simulink model "Xcvr_SSB_AM_2p5"  (Simulink 8.0)
settings: Solver=VariableStepDiscrete  SolverMode=SingleTasking  StartTime=0.0  StopTime=10  RelTol=1e-3
PreLoadFcn:
  | Fs=80e6;
  | 
  | phee=da_rom();
  | [phee_1,phee_2]=da_i2_rom();
  | 
  | Dcic=64;       % CIC decimation
  | Dfac=128;    % following DA filter decimation
  | N = 6;           %       (2^(N+1))=Dfac
  | Daudio=Dcic*Dfac;
  | Faudio=Fs/Daudio;
  | 
  | load info_filt_ssb_4
  | load Serial_Intfc_Stream_5
  | 
  | % AGC related
  | x=0.5:1/256:(1-1/256);
  | addr=(x-0.5)*256;
  | y=1./x;
values from neighbouring files (symbols this model uses):
  Serial_Interface = [0 0 0 0 0 0 0 0 0 0 0 0 ... (11390 elements, 2x5695)]    [Serial_Intfc_Stream_5.mat]
undefined symbols (not defined in the file or in its folder): get, sided, Two, xlipgetpartsetting
undefined symbols (not defined in the file): ssb_coef
libraries: xbsIndex_r4 x1305, dspsrcs4 x5, simulink x2, dspsigops x2, dspsnks4 x1
(part 4 of 11)

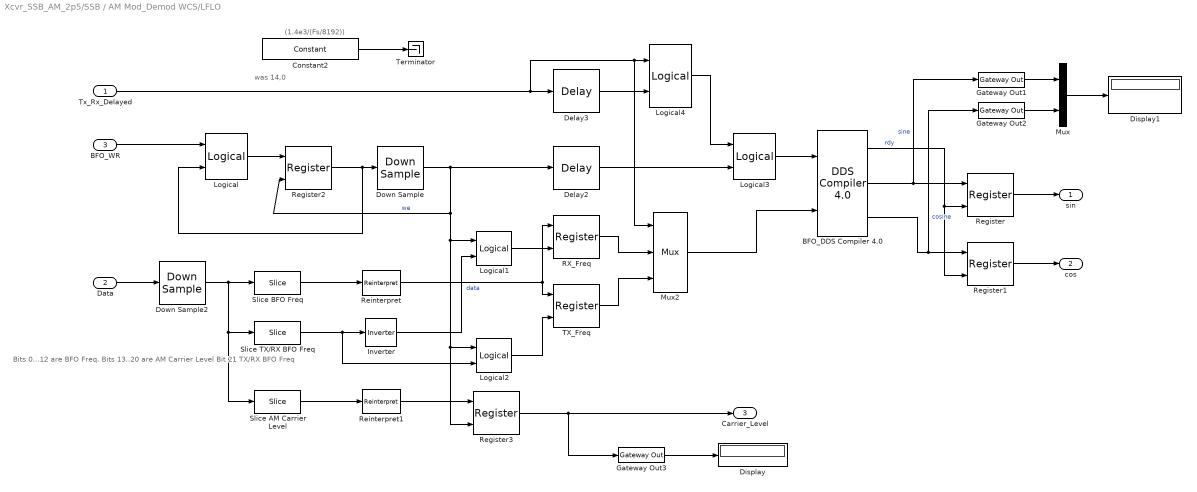
== system Xcvr_SSB_AM_2p5/SSB / AM Mod_Demod WCS/LFLO ==
  note: (1.4e3/(Fs/8192))
  note: was 14,0
  note: Bits 0...12  are BFO Freq.
      | Bits 13..20 are AM Carrier Level
      | Bit 21 TX/RX BFO Freq
  Tx_Rx_Delayed : Inport
  Data : Inport  Port=2
  BFO_WR : Inport  Port=3
  "BFO_DDS Compiler 4.0 " : xbsIndex_r4/DDS Compiler 4.0   partspresent=Phase_Generator_and_SIN_COS_LUT  dds_clock_rate="(Fs/4096)*1e-6 % a LIE  but 8192 does not work!!!!"  channels=1  parameter_entry=System_Parameters  spurious_free_dynamic_range=84  frequency_resolution=(Fs/Daudio)*2^-12  noise_shaping=Phase_Dithering  phase_width=28  output_width=6  output_selection=Sine_and_Cosine  negative_sine=off  negative_cosine=off  amplitude_mode=Full_Range  memory_type=Auto  optimization_goal=Area  dsp48_use=Minimal  latency_configuration=Auto  latency=2  has_phase_out=off  sclr_pin=off  clock_enable=off  rfd=off  rdy=on  channel_pin=off  explicit_period=off  period=1  phase_increment=Programmable  output_frequency1=0  output_frequency2=0  output_frequency3=0  output_frequency4=0  output_frequency5=0  output_frequency6=0  output_frequency7=0  output_frequency8=0  output_frequency9=0  output_frequency10=0  output_frequency11=0  output_frequency12=0  output_frequency13=0  output_frequency14=0  output_frequency15=0  output_frequency16=0  pinc1='0'  pinc2='0'  pinc3='0'  pinc4='0'  pinc5='0'  pinc6='0'  pinc7='0'  pinc8='0'  pinc9='0'  pinc10='0'  pinc11='0'  pinc12='0'  pinc13='0'  pinc14='0'  pinc15='0'  pinc16='0'  phase_offset=None  phase_offset_angles1=0  phase_offset_angles2=0  phase_offset_angles3=0  phase_offset_angles4=0  phase_offset_angles5=0  phase_offset_angles6=0  phase_offset_angles7=0  phase_offset_angles8=0  phase_offset_angles9=0  phase_offset_angles10=0  phase_offset_angles11=0  phase_offset_angles12=0  phase_offset_angles13=0  phase_offset_angles14=0  phase_offset_angles15=0  phase_offset_angles16=0  poff1='0'  poff2='0'  poff3='0'  poff4='0'  poff5='0'  poff6='0'  poff7='0'  poff8='0'  poff9='0'  poff10='0'  poff11='0'  poff12='0'  poff13='0'  poff14='0'  poff15='0'  poff16='0'  por_mode=false  gui_behaviour=Sysgen  ip_name=DDS Compiler  ip_version=4.0  dsptool_ready=true  wrapper_available=true  port_translation_map={ 'ce' => 'en', 'sclr' => 'rst' }  ipcore_xco_need_fpga_part=true  ipcore_fpga_part=xlipgetpartsetting(gcb, {'virtex4', 'xc4vsx35', '-10', 'ff668'})  ipcore_usecache=true  ipcore_useipmodelcache=true  ipcore_verbose=false  block_type=dds_compiler_v4_0
      settings: block_version=12.1
  Constant2 : xbsIndex_r4/Constant  const=(1.4e3/(Fs/8192))  gui_display_data_type=Fixed-point  arith_type=Signed (2's comp)  n_bits=13  bin_pt=13  preci_type=Single  exp_width=8  frac_width=24  explicit_period=on  period=8192/Fs  equ=P=C  opselect=C  inp2=PCIN>>17  opr=+  inp1=P  carry=CIN  dbl_ovrd=off  block_type=constant
      settings: block_version=9.2.00
  Delay2 : xbsIndex_r4/Delay  rst=off  infoeditControl=Selection of Reset will increase slice count due to use of real FFs and instead of SRLs  en=off  latency=1  dbl_ovrd=off  reg_retiming=off  block_type=delay
      settings: block_version=12.1
  Delay3 : xbsIndex_r4/Delay  rst=off  infoeditControl=Selection of Reset will increase slice count due to use of real FFs and instead of SRLs  en=off  latency=1  dbl_ovrd=off  reg_retiming=off  block_type=delay
      settings: block_version=12.1
  Display : Display
  Display1 : Display
  Down Sample : xbsIndex_r4/Down Sample  sample_ratio=1024  sample_phase=First Value of Frame  en=off  latency=0  dbl_ovrd=off  block_type=dsamp
      settings: block_version=9.2.00
  Down Sample2 : xbsIndex_r4/Down Sample  sample_ratio=1024  sample_phase=First Value of Frame  en=off  latency=0  dbl_ovrd=off  block_type=dsamp
      settings: block_version=9.2.00
  Gateway Out1 : xbsIndex_r4/Gateway Out  inherit_from_input=off  hdl_port=off  timing_constraint=None  locs_specified=off  LOCs={}  UseAsDAC=off  DACChannel='1'  block_type=gatewayout
      settings: infoedit="Gateway out block.  Converts Xilinx fixed point inputs into ouputs of type Simulink integer, double, or fixed point.<P><P>Hardware notes:  In hardware these blocks become top level output ports or are discarded, depending on how they are configured."  block_version=9.2.00
  Gateway Out2 : xbsIndex_r4/Gateway Out  inherit_from_input=off  hdl_port=off  timing_constraint=None  locs_specified=off  LOCs={}  UseAsDAC=off  DACChannel='1'  block_type=gatewayout
      settings: infoedit="Gateway out block.  Converts Xilinx fixed point inputs into ouputs of type Simulink integer, double, or fixed point.<P><P>Hardware notes:  In hardware these blocks become top level output ports or are discarded, depending on how they are configured."  block_version=9.2.00
  Gateway Out3 : xbsIndex_r4/Gateway Out  inherit_from_input=off  hdl_port=off  timing_constraint=None  locs_specified=off  LOCs={}  UseAsDAC=off  DACChannel='1'  block_type=gatewayout
      settings: infoedit="Gateway out block.  Converts Xilinx fixed point inputs into ouputs of type Simulink integer, double, or fixed point.<P><P>Hardware notes:  In hardware these blocks become top level output ports or are discarded, depending on how they are configured."  block_version=9.2.00
  Inverter : xbsIndex_r4/Inverter  en=off  latency=0  dbl_ovrd=off  block_type=inv
      settings: block_version=12.2
  Logical : xbsIndex_r4/Logical  logical_function=OR  inputs=2  en=off  latency=0  precision=Full  arith_type=Unsigned  n_bits=16  bin_pt=0  align_bp=on  dbl_ovrd=off  block_type=logical
      settings: block_version=9.2.00
  Logical1 : xbsIndex_r4/Logical  logical_function=AND  inputs=2  en=off  latency=0  precision=Full  arith_type=Unsigned  n_bits=16  bin_pt=0  align_bp=on  dbl_ovrd=off  block_type=logical
      settings: block_version=12.2
  Logical2 : xbsIndex_r4/Logical  logical_function=AND  inputs=2  en=off  latency=0  precision=Full  arith_type=Unsigned  n_bits=16  bin_pt=0  align_bp=on  dbl_ovrd=off  block_type=logical
      settings: block_version=12.2
  Logical3 : xbsIndex_r4/Logical  logical_function=OR  inputs=2  en=off  latency=0  precision=Full  arith_type=Unsigned  n_bits=16  bin_pt=0  align_bp=on  dbl_ovrd=off  block_type=logical
      settings: block_version=12.1
  Logical4 : xbsIndex_r4/Logical  logical_function=XOR  inputs=2  en=off  latency=0  precision=Full  arith_type=Unsigned  n_bits=16  bin_pt=0  align_bp=on  dbl_ovrd=off  block_type=logical
      settings: block_version=12.1
  Mux : Mux  Inputs=2
  Mux2 : xbsIndex_r4/Mux  inputs=2  en=off  latency=0  precision=Full  arith_type=Unsigned  n_bits=16  bin_pt=14  quantization=Truncate  overflow=Wrap  dbl_ovrd=off  block_type=mux
      settings: block_version=12.1
  RX_Freq : xbsIndex_r4/Register  init=0  rst=off  en=on  dbl_ovrd=off  block_type=register
      settings: block_version=12.1
  Register : xbsIndex_r4/Register  init=0  rst=off  en=on  dbl_ovrd=off  block_type=register
      settings: block_version=9.2.00
  Register1 : xbsIndex_r4/Register  init=0  rst=off  en=on  dbl_ovrd=off  block_type=register
      settings: block_version=9.2.00
  Register2 : xbsIndex_r4/Register  init=0  rst=on  en=off  dbl_ovrd=off  block_type=register
      settings: block_version=9.2.00
  Register3 : xbsIndex_r4/Register  init=0.5  rst=off  en=on  dbl_ovrd=off  block_type=register
      settings: block_version=9.2.00
  Reinterpret : xbsIndex_r4/Reinterpret  force_arith_type=on  arith_type="Signed  (2's comp)"  force_bin_pt=on  bin_pt=13  block_type=reinterpret
      settings: infoedit="Changes signal type without altering the binary representation.   You can changed the signal between signed and unsigned, and relocate the binary point.<br><br>Hardware notes: In hardware this block costs nothing.<br><br>Example:  Suppose the input is 6 bits wide, signed, with 2 fractional bits, and the output is forced to unsigned with 0 fractional bits.  Then an input of -2.0 (1110.00 in binary 2's complement) becomes an output of 56 (111000 in binary)."  block_version=9.2.00
  Reinterpret1 : xbsIndex_r4/Reinterpret  force_arith_type=on  arith_type=Unsigned  force_bin_pt=on  bin_pt=8  block_type=reinterpret
      settings: infoedit="Changes signal type without altering the binary representation.   You can changed the signal between signed and unsigned, and relocate the binary point.<br><br>Hardware notes: In hardware this block costs nothing.<br><br>Example:  Suppose the input is 6 bits wide, signed, with 2 fractional bits, and the output is forced to unsigned with 0 fractional bits.  Then an input of -2.0 (1110.00 in binary 2's complement) becomes an output of 56 (111000 in binary)."  block_version=9.2.00
  Slice AM Carrier Level : xbsIndex_r4/Slice  nbits=8  boolean_output=off  mode=Lower Bit Location + Width  bit1=0  base1=MSB of Input  bit0=13  base0=LSB of Input  dbl_ovrd=off  block_type=slice
      settings: block_version=9.2.00
  Slice BFO Freq : xbsIndex_r4/Slice  nbits=13  boolean_output=off  mode=Lower Bit Location + Width  bit1=0  base1=MSB of Input  bit0=0  base0=LSB of Input  dbl_ovrd=off  block_type=slice
      settings: block_version=9.2.00
  Slice TX/RX BFO Freq : xbsIndex_r4/Slice  nbits=1  boolean_output=on  mode=Lower Bit Location + Width  bit1=0  base1=MSB of Input  bit0=21  base0=LSB of Input  dbl_ovrd=off  block_type=slice
      settings: block_version=9.2.00
  TX_Freq : xbsIndex_r4/Register  init=0  rst=off  en=on  dbl_ovrd=off  block_type=register
      settings: block_version=12.1
  Terminator : Terminator
  sin : Outport
  cos : Outport  Port=2
  Carrier_Level : Outport  Port=3
  wires:
  BFO_WR/1 -> Logical/1
  Register/1 -> sin/1
  Register1/1 -> cos/1
  Constant2/1 -> Terminator/1
  Slice BFO Freq/1 -> Reinterpret/1
  Down Sample/1 -> Delay2/1, Register2/2, Logical1/1, Register3/2, Logical2/1  "we"
  Logical/1 -> Register2/1
  Register2/1 -> Logical/2, Down Sample/1
  Gateway Out3/1 -> Display/1
  Data/1 -> Down Sample2/1
  "BFO_DDS Compiler 4.0 "/1 -> Register1/2, Register/2  "rdy"
  "BFO_DDS Compiler 4.0 "/2 -> Register/1, Gateway Out1/1  "sine"
  "BFO_DDS Compiler 4.0 "/3 -> Register1/1, Gateway Out2/1  "cosine"
  Gateway Out1/1 -> Mux/1
  Gateway Out2/1 -> Mux/2
  Mux/1 -> Display1/1
  Slice AM Carrier Level/1 -> Reinterpret1/1
  Reinterpret1/1 -> Register3/1
  Register3/1 -> Carrier_Level/1, Gateway Out3/1
  Down Sample2/1 -> Slice BFO Freq/1, Slice AM Carrier Level/1, Slice TX/RX BFO Freq/1
  Logical3/1 -> "BFO_DDS Compiler 4.0 "/1
  Delay3/1 -> Logical4/2
  Logical4/1 -> Logical3/1
  Delay2/1 -> Logical3/2
  Tx_Rx_Delayed/1 -> Delay3/1, Logical4/1, Mux2/1
  RX_Freq/1 -> Mux2/2
  TX_Freq/1 -> Mux2/3
  Mux2/1 -> "BFO_DDS Compiler 4.0 "/2
  Reinterpret/1 -> RX_Freq/1, TX_Freq/1  "data"
  Slice TX/RX BFO Freq/1 -> Inverter/1, Logical2/2
  Logical1/1 -> RX_Freq/2
  Inverter/1 -> Logical1/2
  Logical2/1 -> TX_Freq/2

== system Xcvr_SSB_AM_2p5/SSB / AM Mod_Demod WCS/Sequential_Complex_abs() ==
  note: Fixed Point Iterative Square Root with Pre/Post Scaling
  In_I : Inport
  In_Q : Inport  Port=2
  AddSub : xbsIndex_r4/AddSub  mode=Addition  use_carryin=off  use_carryout=off  en=off  latency=0  precision=User Defined  arith_type=Unsigned  n_bits=32  bin_pt=31  quantization=Truncate  overflow=Saturate  dbl_ovrd=off  use_behavioral_HDL=off  hw_selection=Fabric  pipelined=off  block_type=addsub
      settings: block_version=12.1
  Convert NOTE Rounding : xbsIndex_r4/Convert  gui_display_data_type=Fixed-point  arith_type="Signed  (2's comp)"  n_bits=18  bin_pt=17  float_type=Single  exp_bits=8  fraction_bits=24  quantization="Round  (unbiased: +/- Inf)"  overflow=Saturate  en=off  latency=0  dbl_ovrd=off  pipeline=off  block_type=convert
      settings: block_version=12.1
  Convert NOTE Rounding1 : xbsIndex_r4/Convert  gui_display_data_type=Fixed-point  arith_type=Unsigned  n_bits=16  bin_pt=15  float_type=Single  exp_bits=8  fraction_bits=24  quantization="Round  (unbiased: +/- Inf)"  overflow=Wrap  en=off  latency=1  dbl_ovrd=off  pipeline=off  block_type=convert
      settings: block_version=12.1
  Delay : xbsIndex_r4/Delay  rst=off  infoeditControl=Selection of Reset will increase slice count due to use of real FFs and instead of SRLs  en=off  latency=1  dbl_ovrd=off  reg_retiming=off  block_type=delay
      settings: block_version=12.1
  Delay1 : xbsIndex_r4/Delay  rst=off  infoeditControl=Selection of Reset will increase slice count due to use of real FFs and instead of SRLs  en=off  latency=1  dbl_ovrd=off  reg_retiming=off  block_type=delay
      settings: block_version=12.1
  Down Sample : xbsIndex_r4/Down Sample  sample_ratio=32  sample_phase="Last Value of Frame  (most efficient)"  en=off  latency=1  dbl_ovrd=off  block_type=dsamp
      settings: block_version=12.1
  Iterative SQRT : Subsystem
  Pre Scaler : Subsystem
  Sequential Post Scale : Subsystem
  Time Shared Square Operator : Subsystem
  Up Sample : xbsIndex_r4/Up Sample  sample_ratio=32  copy_samples=on  en=off  latency=0  dbl_ovrd=off  block_type=usamp
      settings: block_version=12.1
  Up Sample1 : xbsIndex_r4/Up Sample  sample_ratio=32  copy_samples=on  en=off  latency=0  dbl_ovrd=off  block_type=usamp
      settings: block_version=12.1
  Out1 : Outport
  wires:
  Iterative SQRT/2("To SQR ") -> Convert NOTE Rounding/1
  Pre Scaler/1(X*(2^2n)) -> Iterative SQRT/1(Xin)
  Pre Scaler/2(Done) -> Iterative SQRT/2(Run)  "RUN"
  Up Sample/1 -> Time Shared Square Operator/1(A)
  Time Shared Square Operator/2(B^2) -> AddSub/2
  Time Shared Square Operator/1(A^2) -> AddSub/1
  In_I/1 -> Delay/1
  In_Q/1 -> Delay1/1
  Up Sample1/1 -> Time Shared Square Operator/2(B)
  Time Shared Square Operator/3(C^2) -> Iterative SQRT/3(From SQR)
  AddSub/1 -> Pre Scaler/1(X)
  Convert NOTE Rounding/1 -> Time Shared Square Operator/3(C)
  Iterative SQRT/1(Raw Sqrt Out) -> Sequential Post Scale/1(X)  "RAW Sqrt"
  Convert NOTE Rounding1/1 -> Out1/1
  Delay/1 -> Up Sample/1
  Delay1/1 -> Up Sample1/1
  Pre Scaler/3(Shift Count) -> Down Sample/1  "Shift"
  Down Sample/1 -> Sequential Post Scale/2(n)
  Sequential Post Scale/1(X*(2^-n)) -> Convert NOTE Rounding1/1

== system Xcvr_SSB_AM_2p5/SSB / AM Mod_Demod WCS/Time_Share_MPY ==
  note: An even number of Mults is needed.
  A : Inport
  a : Inport  Port=2
  B : Inport  Port=3
  b : Inport  Port=4
  C : Inport  Port=5
  c : Inport  Port=6
  D : Inport  Port=7
  d : Inport  Port=8
  Mult2 : xbsIndex_r4/Mult  precision=User Defined  arith_type="Signed  (2's comp)"  n_bits=18  bin_pt=17  quantization="Round  (unbiased: +/- Inf)"  overflow=Saturate  en=off  latency=4  dbl_ovrd=off  use_behavioral_HDL=off  opt=Area  use_embedded=on  optimum_pipeline=off  pipeline=on  use_rpm=on  placement_style=Triangular  block_type=mult
      settings: block_version=9.2.00
  Time Division Demultiplexer : xbsIndex_r4/Time Division Demultiplexer  frame_pattern=[1 1 1 1]  impl_style=Multiple Channel  vin=off  dbl_ovrd=off  explicit_period=off  period=1  block_type=tdd
      settings: infoedit=Samples presented at the input are selected and down-sampled according to the frame sampling pattern specified. The sampled input is presented either as a single or multiple channel at the output.  block_version=12.1
  Time Division Multiplexer : xbsIndex_r4/Time Division Multiplexer  inputs=4  vin=off  dbl_ovrd=off  explicit_period=off  period=1  block_type=tdm
      settings: infoedit="Multiple inputs are sampled and  presented serially at the output."
  Time Division Multiplexer1 : xbsIndex_r4/Time Division Multiplexer  inputs=4  vin=off  dbl_ovrd=off  explicit_period=off  period=1  block_type=tdm
      settings: infoedit="Multiple inputs are sampled and  presented serially at the output."
  A*a : Outport
  B*b : Outport  Port=2
  C*c : Outport  Port=3
  D*d : Outport  Port=4
  wires:
  Time Division Multiplexer/1 -> Mult2/1
  Mult2/1 -> Time Division Demultiplexer/1
  A/1 -> Time Division Multiplexer/1
  B/1 -> Time Division Multiplexer/2
  Time Division Demultiplexer/1 -> A*a/1
  Time Division Demultiplexer/2 -> B*b/1
  Time Division Demultiplexer/3 -> C*c/1
  Time Division Demultiplexer/4 -> D*d/1
  a/1 -> Time Division Multiplexer1/1
  b/1 -> Time Division Multiplexer1/2
  c/1 -> Time Division Multiplexer1/3
  d/1 -> Time Division Multiplexer1/4
  Time Division Multiplexer1/1 -> Mult2/2
  C/1 -> Time Division Multiplexer/3
  D/1 -> Time Division Multiplexer/4

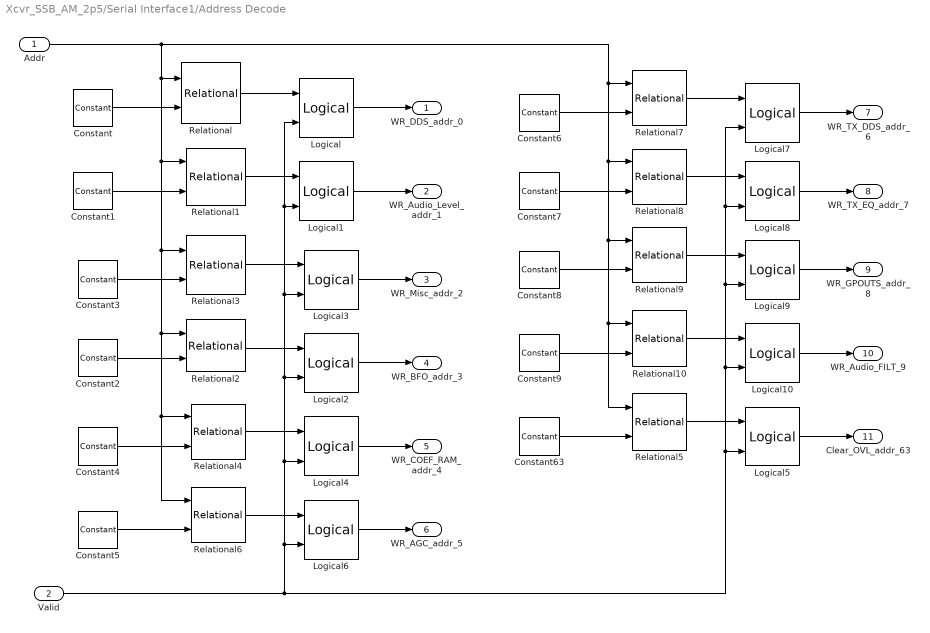
== system Xcvr_SSB_AM_2p5/Serial Interface1/Address Decode ==
  Addr : Inport
  Valid : Inport  Port=2
  Constant : xbsIndex_r4/Constant  const=0  gui_display_data_type=Fixed-point  arith_type=Unsigned  n_bits=6  bin_pt=0  preci_type=Single  exp_width=8  frac_width=24  explicit_period=off  period=1  equ=P=C  opselect=C  inp2=PCIN>>17  opr=+  inp1=P  carry=CIN  dbl_ovrd=off  block_type=constant
      settings: block_version=9.2.00
  Constant1 : xbsIndex_r4/Constant  const=1  gui_display_data_type=Fixed-point  arith_type=Unsigned  n_bits=6  bin_pt=0  preci_type=Single  exp_width=8  frac_width=24  explicit_period=off  period=1  equ=P=C  opselect=C  inp2=PCIN>>17  opr=+  inp1=P  carry=CIN  dbl_ovrd=off  block_type=constant
      settings: block_version=9.2.00
  Constant2 : xbsIndex_r4/Constant  const=3  gui_display_data_type=Fixed-point  arith_type=Unsigned  n_bits=6  bin_pt=0  preci_type=Single  exp_width=8  frac_width=24  explicit_period=off  period=1  equ=P=C  opselect=C  inp2=PCIN>>17  opr=+  inp1=P  carry=CIN  dbl_ovrd=off  block_type=constant
      settings: block_version=9.2.00
  Constant3 : xbsIndex_r4/Constant  const=2  gui_display_data_type=Fixed-point  arith_type=Unsigned  n_bits=6  bin_pt=0  preci_type=Single  exp_width=8  frac_width=24  explicit_period=off  period=1  equ=P=C  opselect=C  inp2=PCIN>>17  opr=+  inp1=P  carry=CIN  dbl_ovrd=off  block_type=constant
      settings: block_version=9.2.00
  Constant4 : xbsIndex_r4/Constant  const=4  gui_display_data_type=Fixed-point  arith_type=Unsigned  n_bits=6  bin_pt=0  preci_type=Single  exp_width=8  frac_width=24  explicit_period=off  period=1  equ=P=C  opselect=C  inp2=PCIN>>17  opr=+  inp1=P  carry=CIN  dbl_ovrd=off  block_type=constant
      settings: block_version=9.2.00
  Constant5 : xbsIndex_r4/Constant  const=5  gui_display_data_type=Fixed-point  arith_type=Unsigned  n_bits=6  bin_pt=0  preci_type=Single  exp_width=8  frac_width=24  explicit_period=off  period=1  equ=P=C  opselect=C  inp2=PCIN>>17  opr=+  inp1=P  carry=CIN  dbl_ovrd=off  block_type=constant
      settings: block_version=9.2.00
  Constant6 : xbsIndex_r4/Constant  const=6  gui_display_data_type=Fixed-point  arith_type=Unsigned  n_bits=6  bin_pt=0  preci_type=Single  exp_width=8  frac_width=24  explicit_period=off  period=1  equ=P=C  opselect=C  inp2=PCIN>>17  opr=+  inp1=P  carry=CIN  dbl_ovrd=off  block_type=constant
      settings: block_version=9.2.00
  Constant63 : xbsIndex_r4/Constant  const=63  gui_display_data_type=Fixed-point  arith_type=Unsigned  n_bits=6  bin_pt=0  preci_type=Single  exp_width=8  frac_width=24  explicit_period=off  period=1  equ=P=C  opselect=C  inp2=PCIN>>17  opr=+  inp1=P  carry=CIN  dbl_ovrd=off  block_type=constant
      settings: block_version=9.2.00
  Constant7 : xbsIndex_r4/Constant  const=7  gui_display_data_type=Fixed-point  arith_type=Unsigned  n_bits=6  bin_pt=0  preci_type=Single  exp_width=8  frac_width=24  explicit_period=off  period=1  equ=P=C  opselect=C  inp2=PCIN>>17  opr=+  inp1=P  carry=CIN  dbl_ovrd=off  block_type=constant
      settings: block_version=9.2.00
  Constant8 : xbsIndex_r4/Constant  const=8  gui_display_data_type=Fixed-point  arith_type=Unsigned  n_bits=6  bin_pt=0  preci_type=Single  exp_width=8  frac_width=24  explicit_period=off  period=1  equ=P=C  opselect=C  inp2=PCIN>>17  opr=+  inp1=P  carry=CIN  dbl_ovrd=off  block_type=constant
      settings: block_version=9.2.00
  Constant9 : xbsIndex_r4/Constant  const=9  gui_display_data_type=Fixed-point  arith_type=Unsigned  n_bits=6  bin_pt=0  preci_type=Single  exp_width=8  frac_width=24  explicit_period=off  period=1  equ=P=C  opselect=C  inp2=PCIN>>17  opr=+  inp1=P  carry=CIN  dbl_ovrd=off  block_type=constant
      settings: block_version=9.2.00
  Logical{,1..10} (11 alike) : xbsIndex_r4/Logical  logical_function=AND  inputs=2  en=off  latency=0  precision=Full  arith_type=Unsigned  n_bits=16  bin_pt=0  align_bp=on  dbl_ovrd=off  block_type=logical
      settings: block_version=9.2.00
  Relational{,1..10} (11 alike) : xbsIndex_r4/Relational  mode=a=b  en=off  latency=0  dbl_ovrd=off  block_type=relational
      settings: block_version=9.2.00
  WR_DDS_addr_0 : Outport
  WR_Audio_Level_addr_1 : Outport  Port=2
  WR_Misc_addr_2 : Outport  Port=3
  WR_BFO_addr_3 : Outport  Port=4
  WR_COEF_RAM_addr_4 : Outport  Port=5
  WR_AGC_addr_5 : Outport  Port=6
  WR_TX_DDS_addr_6 : Outport  Port=7
  WR_TX_EQ_addr_7 : Outport  Port=8
  WR_GPOUTS_addr_8 : Outport  Port=9
  WR_Audio_FILT_9 : Outport  Port=10
  Clear_OVL_addr_63 : Outport  Port=11
  wires:
  Constant/1 -> Relational/2
  Addr/1 -> Relational/1, Relational1/1, Relational3/1, Relational2/1, Relational4/1, Relational6/1, Relational7/1, Relational8/1, Relational5/1, Relational10/1, Relational9/1
  Constant1/1 -> Relational1/2
  Relational/1 -> Logical/1
  Logical/1 -> WR_DDS_addr_0/1
  Logical1/1 -> WR_Audio_Level_addr_1/1
  Relational1/1 -> Logical1/1
  Constant2/1 -> Relational2/2
  Logical2/1 -> WR_BFO_addr_3/1
  Relational2/1 -> Logical2/1
  Constant3/1 -> Relational3/2
  Relational3/1 -> Logical3/1
  Logical3/1 -> WR_Misc_addr_2/1
  Constant4/1 -> Relational4/2
  Logical4/1 -> WR_COEF_RAM_addr_4/1
  Relational4/1 -> Logical4/1
  Constant5/1 -> Relational6/2
  Relational6/1 -> Logical6/1
  Logical6/1 -> WR_AGC_addr_5/1
  Logical10/1 -> WR_Audio_FILT_9/1
  Valid/1 -> Logical5/2, Logical10/2, Logical9/2, Logical7/2, Logical8/2, Logical6/2, Logical4/2, Logical2/2, Logical3/2, Logical/2, Logical1/2
  Constant63/1 -> Relational5/2
  Relational5/1 -> Logical5/1
  Logical5/1 -> Clear_OVL_addr_63/1
  Relational7/1 -> Logical7/1
  Constant6/1 -> Relational7/2
  Logical7/1 -> WR_TX_DDS_addr_6/1
  Constant7/1 -> Relational8/2
  Relational8/1 -> Logical8/1
  Logical8/1 -> WR_TX_EQ_addr_7/1
  Relational9/1 -> Logical9/1
  Logical9/1 -> WR_GPOUTS_addr_8/1
  Constant8/1 -> Relational9/2
  Constant9/1 -> Relational10/2
  Relational10/1 -> Logical10/1

== system Xcvr_SSB_AM_2p5/Serial Interface1/GP_Outputs ==
  Reg_Data : Inport
  WR_GP_REG : Inport  Port=2
  Data_0 : xbsIndex_r4/Slice  nbits=1  boolean_output=on  mode=Lower Bit Location + Width  bit1=-3  base1=MSB of Input  bit0=0  base0=LSB of Input  dbl_ovrd=off  block_type=slice
      settings: block_version=9.2.00
  Data_15-1 : xbsIndex_r4/Slice  nbits=15  boolean_output=off  mode=Lower Bit Location + Width  bit1=-2  base1=MSB of Input  bit0=1  base0=LSB of Input  dbl_ovrd=off  block_type=slice
      settings: block_version=9.2.00
  Data_24-20 : xbsIndex_r4/Slice  nbits=5  boolean_output=off  mode=Lower Bit Location + Width  bit1=-2  base1=MSB of Input  bit0=20  base0=LSB of Input  dbl_ovrd=off  block_type=slice
      settings: block_version=9.2.00
  Data_25 : xbsIndex_r4/Slice  nbits=1  boolean_output=on  mode=Lower Bit Location + Width  bit1=-3  base1=MSB of Input  bit0=25  base0=LSB of Input  dbl_ovrd=off  block_type=slice
      settings: block_version=9.2.00
  Down Sample1 : xbsIndex_r4/Down Sample  sample_ratio=1024  sample_phase="Last Value of Frame  (most efficient)"  en=off  latency=1  dbl_ovrd=off  block_type=dsamp
      settings: block_version=9.2.00
  Down Sample2 : xbsIndex_r4/Down Sample  sample_ratio=1024  sample_phase="Last Value of Frame  (most efficient)"  en=off  latency=1  dbl_ovrd=off  block_type=dsamp
      settings: block_version=9.2.00
  Down Sample3 : xbsIndex_r4/Down Sample  sample_ratio=1024  sample_phase="Last Value of Frame  (most efficient)"  en=off  latency=1  dbl_ovrd=off  block_type=dsamp
      settings: block_version=9.2.00
  Register1 : xbsIndex_r4/Register  init=0  rst=off  en=on  dbl_ovrd=off  block_type=register
      settings: block_version=9.2.00
  GP_OUT_BIT_1_to15 : Outport
  P23_SEL : Outport  Port=2
  IRPT_EN_0to4 : Outport  Port=3
  EN_EXT_PA_TR : Outport  Port=4
  wires:
  Reg_Data/1 -> Register1/1
  WR_GP_REG/1 -> Register1/2
  Down Sample1/1 -> GP_OUT_BIT_1_to15/1
  Data_15-1/1 -> Down Sample1/1
  Data_24-20/1 -> IRPT_EN_0to4/1
  Down Sample2/1 -> P23_SEL/1
  Data_25/1 -> Down Sample2/1
  Register1/1 -> Data_25/1, Data_24-20/1, Data_15-1/1, Data_0/1
  Data_0/1 -> Down Sample3/1
  Down Sample3/1 -> EN_EXT_PA_TR/1

== system Xcvr_SSB_AM_2p5/Serial Interface1/Interrupt_Generator ==
  note: Interrupts:
      | 0 - DIN0
      | 1 - DIN1
      | 2 - DIN2
      | 3 - DIN3
      | 4 - nOVLD
  note: Logic running at 10 MHz
  IRPT_EN_0to4 : Inport
  CLR_IRPTS : Inport  Port=2
  DIN_0to3 : Inport  Port=3
  nOVLD : Inport  Port=4
  Concat : xbsIndex_r4/Concat  num_inputs=5  dbl_ovrd=off  block_type=concat
      settings: block_version=12.1
  IRPT_REG0 : Subsystem
  IRPT_REG1 : Subsystem
  IRPT_REG2 : Subsystem
  IRPT_REG3 : Subsystem
  IRPT_REG4 : Subsystem
  Logical2 : xbsIndex_r4/Logical  logical_function=OR  inputs=5  en=off  latency=0  precision=Full  arith_type=Unsigned  n_bits=16  bin_pt=0  align_bp=on  dbl_ovrd=off  block_type=logical
      settings: block_version=12.1
  Slice0 : xbsIndex_r4/Slice  nbits=1  boolean_output=on  mode=Lower Bit Location + Width  bit1=0  base1=MSB of Input  bit0=0  base0=LSB of Input  dbl_ovrd=off  block_type=slice
      settings: block_version=12.1
  Slice1 : xbsIndex_r4/Slice  nbits=1  boolean_output=on  mode=Lower Bit Location + Width  bit1=0  base1=MSB of Input  bit0=1  base0=LSB of Input  dbl_ovrd=off  block_type=slice
      settings: block_version=12.1
  Slice2 : xbsIndex_r4/Slice  nbits=1  boolean_output=on  mode=Lower Bit Location + Width  bit1=0  base1=MSB of Input  bit0=2  base0=LSB of Input  dbl_ovrd=off  block_type=slice
      settings: block_version=12.1
  Slice3 : xbsIndex_r4/Slice  nbits=1  boolean_output=on  mode=Lower Bit Location + Width  bit1=0  base1=MSB of Input  bit0=3  base0=LSB of Input  dbl_ovrd=off  block_type=slice
      settings: block_version=12.1
  Slice4 : xbsIndex_r4/Slice  nbits=1  boolean_output=on  mode=Lower Bit Location + Width  bit1=0  base1=MSB of Input  bit0=0  base0=LSB of Input  dbl_ovrd=off  block_type=slice
      settings: block_version=12.1
  Slice5 : xbsIndex_r4/Slice  nbits=1  boolean_output=on  mode=Lower Bit Location + Width  bit1=0  base1=MSB of Input  bit0=1  base0=LSB of Input  dbl_ovrd=off  block_type=slice
      settings: block_version=12.1
  Slice6 : xbsIndex_r4/Slice  nbits=1  boolean_output=on  mode=Lower Bit Location + Width  bit1=0  base1=MSB of Input  bit0=2  base0=LSB of Input  dbl_ovrd=off  block_type=slice
      settings: block_version=12.1
  Slice7 : xbsIndex_r4/Slice  nbits=1  boolean_output=on  mode=Lower Bit Location + Width  bit1=0  base1=MSB of Input  bit0=3  base0=LSB of Input  dbl_ovrd=off  block_type=slice
      settings: block_version=12.1
  Slice8 : xbsIndex_r4/Slice  nbits=1  boolean_output=on  mode=Lower Bit Location + Width  bit1=0  base1=MSB of Input  bit0=4  base0=LSB of Input  dbl_ovrd=off  block_type=slice
      settings: block_version=12.1
  IRPT_0to4 : Outport
  IRPT : Outport  Port=2
  wires:
  Slice0/1 -> IRPT_REG0/1(DIN)
  Slice1/1 -> IRPT_REG1/1(DIN)
  Slice3/1 -> IRPT_REG3/1(DIN)
  Slice2/1 -> IRPT_REG2/1(DIN)
  Slice4/1 -> IRPT_REG0/2(EN_IRPT)
  Slice5/1 -> IRPT_REG1/2(EN_IRPT)
  Slice6/1 -> IRPT_REG2/2(EN_IRPT)
  Slice7/1 -> IRPT_REG3/2(EN_IRPT)
  Slice8/1 -> IRPT_REG4/2(EN_IRPT)
  DIN_0to3/1 -> Slice0/1, Slice1/1, Slice2/1, Slice3/1
  IRPT_EN_0to4/1 -> Slice8/1, Slice4/1, Slice5/1, Slice6/1, Slice7/1
  CLR_IRPTS/1 -> IRPT_REG0/3(CLR_IRPT), IRPT_REG1/3(CLR_IRPT), IRPT_REG2/3(CLR_IRPT), IRPT_REG3/3(CLR_IRPT), IRPT_REG4/3(CLR_IRPT)
  Logical2/1 -> IRPT/1
  IRPT_REG0/1(IRPT_OUT) -> Logical2/1, Concat/5
  IRPT_REG1/1(IRPT_OUT) -> Logical2/2, Concat/4
  IRPT_REG2/1(IRPT_OUT) -> Logical2/3, Concat/3
  IRPT_REG3/1(IRPT_OUT) -> Logical2/4, Concat/2
  IRPT_REG4/1(IRPT_OUT) -> Logical2/5, Concat/1
  Concat/1 -> IRPT_0to4/1
  nOVLD/1 -> IRPT_REG4/1(DIN)

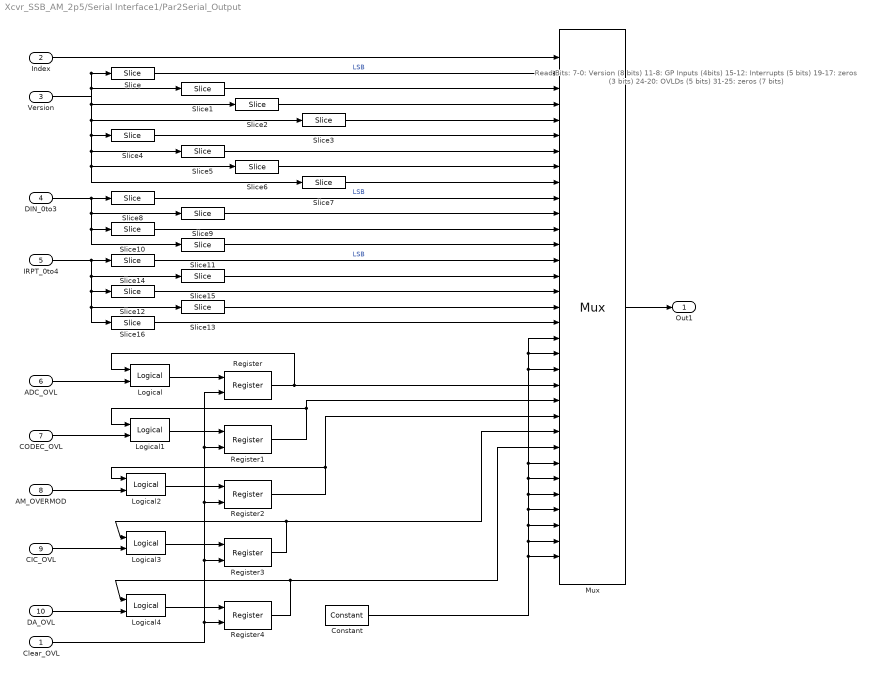
== system Xcvr_SSB_AM_2p5/Serial Interface1/Par2Serial_Output ==
  note: Read Bits:
      |
      | 7-0: Version (8 bits)
      | 11-8: GP Inputs (4bits)
      | 15-12: Interrupts (5 bits)
      | 19-17: zeros (3 bits)
      | 24-20: OVLDs (5 bits)
      | 31-25: zeros (7 bits)
  Clear_OVL : Inport
  Index : Inport  Port=2
  Version : Inport  Port=3
  DIN_0to3 : Inport  Port=4
  IRPT_0to4 : Inport  Port=5
  ADC_OVL : Inport  Port=6
  CODEC_OVL : Inport  Port=7
  AM_OVERMOD : Inport  Port=8
  CIC_OVL : Inport  Port=9
  DA_OVL : Inport  Port=10
  Constant : xbsIndex_r4/Constant  const=0  gui_display_data_type=Fixed-point  arith_type=Boolean  n_bits=16  bin_pt=14  preci_type=Single  exp_width=8  frac_width=24  explicit_period=off  period=1  equ=P=C  opselect=C  inp2=PCIN>>17  opr=+  inp1=P  carry=CIN  dbl_ovrd=off  block_type=constant
      settings: block_version=12.1
  Logical{,1..4} (5 alike) : xbsIndex_r4/Logical  logical_function=OR  inputs=2  en=off  latency=0  precision=Full  arith_type=Unsigned  n_bits=16  bin_pt=0  align_bp=on  dbl_ovrd=off  block_type=logical
      settings: block_version=12.1
  Mux : xbsIndex_r4/Mux  inputs=32  en=off  latency=0  precision=Full  arith_type=Unsigned  n_bits=16  bin_pt=14  quantization=Truncate  overflow=Wrap  dbl_ovrd=off  block_type=mux
      settings: block_version=12.1
  Register{,1..4} (5 alike) : xbsIndex_r4/Register  init=0  rst=on  en=off  dbl_ovrd=off  block_type=register
      settings: block_version=12.1
  Slice : xbsIndex_r4/Slice  nbits=1  boolean_output=on  mode=Lower Bit Location + Width  bit1=0  base1=MSB of Input  bit0=0  base0=LSB of Input  dbl_ovrd=off  block_type=slice
      settings: block_version=12.1
  Slice1 : xbsIndex_r4/Slice  nbits=1  boolean_output=on  mode=Lower Bit Location + Width  bit1=0  base1=MSB of Input  bit0=1  base0=LSB of Input  dbl_ovrd=off  block_type=slice
      settings: block_version=12.1
  Slice10 : xbsIndex_r4/Slice  nbits=1  boolean_output=on  mode=Lower Bit Location + Width  bit1=0  base1=MSB of Input  bit0=2  base0=LSB of Input  dbl_ovrd=off  block_type=slice
      settings: block_version=12.1
  Slice11 : xbsIndex_r4/Slice  nbits=1  boolean_output=on  mode=Lower Bit Location + Width  bit1=0  base1=MSB of Input  bit0=3  base0=LSB of Input  dbl_ovrd=off  block_type=slice
      settings: block_version=12.1
  Slice12 : xbsIndex_r4/Slice  nbits=1  boolean_output=on  mode=Lower Bit Location + Width  bit1=0  base1=MSB of Input  bit0=2  base0=LSB of Input  dbl_ovrd=off  block_type=slice
      settings: block_version=12.1
  Slice13 : xbsIndex_r4/Slice  nbits=1  boolean_output=on  mode=Lower Bit Location + Width  bit1=0  base1=MSB of Input  bit0=3  base0=LSB of Input  dbl_ovrd=off  block_type=slice
      settings: block_version=12.1
  Slice14 : xbsIndex_r4/Slice  nbits=1  boolean_output=on  mode=Lower Bit Location + Width  bit1=0  base1=MSB of Input  bit0=0  base0=LSB of Input  dbl_ovrd=off  block_type=slice
      settings: block_version=12.1
  Slice15 : xbsIndex_r4/Slice  nbits=1  boolean_output=on  mode=Lower Bit Location + Width  bit1=0  base1=MSB of Input  bit0=1  base0=LSB of Input  dbl_ovrd=off  block_type=slice
      settings: block_version=12.1
  Slice16 : xbsIndex_r4/Slice  nbits=1  boolean_output=on  mode=Lower Bit Location + Width  bit1=0  base1=MSB of Input  bit0=4  base0=LSB of Input  dbl_ovrd=off  block_type=slice
      settings: block_version=12.1
  Slice2 : xbsIndex_r4/Slice  nbits=1  boolean_output=on  mode=Lower Bit Location + Width  bit1=0  base1=MSB of Input  bit0=2  base0=LSB of Input  dbl_ovrd=off  block_type=slice
      settings: block_version=12.1
  Slice3 : xbsIndex_r4/Slice  nbits=1  boolean_output=on  mode=Lower Bit Location + Width  bit1=0  base1=MSB of Input  bit0=3  base0=LSB of Input  dbl_ovrd=off  block_type=slice
      settings: block_version=12.1
  Slice4 : xbsIndex_r4/Slice  nbits=1  boolean_output=on  mode=Lower Bit Location + Width  bit1=0  base1=MSB of Input  bit0=4  base0=LSB of Input  dbl_ovrd=off  block_type=slice
      settings: block_version=12.1
  Slice5 : xbsIndex_r4/Slice  nbits=1  boolean_output=on  mode=Lower Bit Location + Width  bit1=0  base1=MSB of Input  bit0=5  base0=LSB of Input  dbl_ovrd=off  block_type=slice
      settings: block_version=12.1
  Slice6 : xbsIndex_r4/Slice  nbits=1  boolean_output=on  mode=Lower Bit Location + Width  bit1=0  base1=MSB of Input  bit0=6  base0=LSB of Input  dbl_ovrd=off  block_type=slice
      settings: block_version=12.1
  Slice7 : xbsIndex_r4/Slice  nbits=1  boolean_output=on  mode=Lower Bit Location + Width  bit1=0  base1=MSB of Input  bit0=7  base0=LSB of Input  dbl_ovrd=off  block_type=slice
      settings: block_version=12.1
  Slice8 : xbsIndex_r4/Slice  nbits=1  boolean_output=on  mode=Lower Bit Location + Width  bit1=0  base1=MSB of Input  bit0=0  base0=LSB of Input  dbl_ovrd=off  block_type=slice
      settings: block_version=12.1
  Slice9 : xbsIndex_r4/Slice  nbits=1  boolean_output=on  mode=Lower Bit Location + Width  bit1=0  base1=MSB of Input  bit0=1  base0=LSB of Input  dbl_ovrd=off  block_type=slice
      settings: block_version=12.1
  Out1 : Outport
  wires:
  Index/1 -> Mux/1
  Mux/1 -> Out1/1
  Version/1 -> Slice/1, Slice1/1, Slice2/1, Slice3/1, Slice4/1, Slice5/1, Slice6/1, Slice7/1
  Slice/1 -> Mux/2  "LSB"
  Slice1/1 -> Mux/3
  Slice2/1 -> Mux/4
  Slice3/1 -> Mux/5
  Slice4/1 -> Mux/6
  Slice5/1 -> Mux/7
  Slice6/1 -> Mux/8
  Slice7/1 -> Mux/9
  Slice8/1 -> Mux/10  "LSB"
  Slice9/1 -> Mux/11
  Slice10/1 -> Mux/12
  Slice11/1 -> Mux/13
  DIN_0to3/1 -> Slice8/1, Slice9/1, Slice10/1, Slice11/1
  Logical/1 -> Register/1
  Register/1 -> Logical/1, Mux/22
  ADC_OVL/1 -> Logical/2
  Clear_OVL/1 -> Register/2, Register1/2, Register2/2, Register3/2, Register4/2
  Logical1/1 -> Register1/1
  Register1/1 -> Logical1/1, Mux/23
  CODEC_OVL/1 -> Logical1/2
  Constant/1 -> Mux/33, Mux/21, Mux/20, Mux/19, Mux/27, Mux/28, Mux/29, Mux/30, Mux/31, Mux/32
  Register2/1 -> Mux/24, Logical2/1
  Logical2/1 -> Register2/1
  AM_OVERMOD/1 -> Logical2/2
  Logical3/1 -> Register3/1
  CIC_OVL/1 -> Logical3/2
  Register3/1 -> Logical3/1, Mux/25
  Logical4/1 -> Register4/1
  Register4/1 -> Logical4/1, Mux/26
  DA_OVL/1 -> Logical4/2
  Slice14/1 -> Mux/14  "LSB"
  Slice12/1 -> Mux/16
  Slice15/1 -> Mux/15
  Slice13/1 -> Mux/17
  Slice16/1 -> Mux/18
  IRPT_0to4/1 -> Slice14/1, Slice15/1, Slice12/1, Slice13/1, Slice16/1

== system Xcvr_SSB_AM_2p5/Serial Interface1/Serial_in_Parallel_out ==
  Sin : Inport
  Clk : Inport  Port=2
  nRST : Inport  Port=3
  26_MSBs : xbsIndex_r4/Slice  nbits=26  boolean_output=off  mode=Upper Bit Location + Width  bit1=0  base1=MSB of Input  bit0=0  base0=LSB of Input  dbl_ovrd=off  block_type=slice
      settings: infoedit="Extracts a given range of bits from each input sample and presents it at the output.  The output type is ordinarily unsigned with binary point at zero, but can be Boolean when the slice is one bit wide.<P><P>Hardware notes: In hardware this block costs nothing."  block_version=9.2.00
  6_LSBs : xbsIndex_r4/Slice  nbits=6  boolean_output=off  mode=Lower Bit Location + Width  bit1=-25  base1=MSB of Input  bit0=0  base0=LSB of Input  dbl_ovrd=off  block_type=slice
      settings: infoedit="Extracts a given range of bits from each input sample and presents it at the output.  The output type is ordinarily unsigned with binary point at zero, but can be Boolean when the slice is one bit wide.<P><P>Hardware notes: In hardware this block costs nothing."  block_version=9.2.00
  Constant : xbsIndex_r4/Constant  const=0  gui_display_data_type=Fixed-point  arith_type=Unsigned  n_bits=5  bin_pt=0  preci_type=Single  exp_width=8  frac_width=24  explicit_period=off  period=1  equ=P=C  opselect=C  inp2=PCIN>>17  opr=+  inp1=P  carry=CIN  dbl_ovrd=off  block_type=constant
      settings: block_version=9.2.00
  Convert : xbsIndex_r4/Convert  gui_display_data_type=Fixed-point  arith_type="Signed  (2's comp)"  n_bits=26  bin_pt=0  float_type=Single  exp_bits=8  fraction_bits=24  quantization=Truncate  overflow=Wrap  en=off  latency=0  dbl_ovrd=off  pipeline=off  block_type=convert
      settings: block_version=9.2.00
  Counter : xbsIndex_r4/Counter  cnt_type=Free Running  cnt_to=Inf  operation=Up  start_count=0  cnt_by_val=1  arith_type=Unsigned  n_bits=5  bin_pt=0  load_pin=off  rst=on  en=on  explicit_period=off  period=1  dbl_ovrd=off  use_behavioral_HDL=off  implementation=Fabric  use_rpm=off  block_type=counter
      settings: block_version=9.2.00
  Delay1 : xbsIndex_r4/Delay  rst=off  infoeditControl=Selection of Reset will increase slice count due to use of real FFs and instead of SRLs  en=off  latency=1  dbl_ovrd=off  reg_retiming=off  block_type=delay
      settings: block_version=9.2.00
  Delay2 : xbsIndex_r4/Delay  rst=off  infoeditControl=Selection of Reset will increase slice count due to use of real FFs and instead of SRLs  en=off  latency=1  dbl_ovrd=off  reg_retiming=off  block_type=delay
      settings: block_version=9.2.00
  Delay3 : xbsIndex_r4/Delay  rst=off  infoeditControl=Selection of Reset will increase slice count due to use of real FFs and instead of SRLs  en=off  latency=1  dbl_ovrd=off  reg_retiming=off  block_type=delay
      settings: block_version=9.2.00
  Inverter : xbsIndex_r4/Inverter  en=off  latency=0  dbl_ovrd=off  block_type=inv
      settings: block_version=12.1
  Logical : xbsIndex_r4/Logical  logical_function=AND  inputs=2  en=off  latency=0  precision=Full  arith_type=Unsigned  n_bits=16  bin_pt=0  align_bp=on  dbl_ovrd=off  block_type=logical
      settings: block_version=12.1
  Logical1 : xbsIndex_r4/Logical  logical_function=OR  inputs=2  en=off  latency=0  precision=Full  arith_type=Unsigned  n_bits=16  bin_pt=0  align_bp=on  dbl_ovrd=off  block_type=logical
      settings: block_version=12.1
  Register : xbsIndex_r4/Register  init=0  rst=off  en=on  dbl_ovrd=off  block_type=register
      settings: block_version=9.2.00
  Register1 : xbsIndex_r4/Register  init=0  rst=off  en=on  dbl_ovrd=off  block_type=register
      settings: block_version=9.2.00
  Relational : xbsIndex_r4/Relational  mode=a=b  en=off  latency=1  dbl_ovrd=off  block_type=relational
      settings: block_version=9.2.00
  Serial2Par : Subsystem
  delta_1 : Subsystem
  delta_2 : Subsystem
  Par_26 : Outport
  Address_6 : Outport  Port=2
  Valid : Outport  Port=3
  RFD : Outport  Port=4
  Index : Outport  Port=5
  wires:
  delta_1/1(Out1) -> Serial2Par/2(ena), Logical1/1
  Counter/1 -> Relational/1, Index/1
  Constant/1 -> Relational/2
  Sin/1 -> Delay2/1
  Serial2Par/1(out_32b) -> 26_MSBs/1, 6_LSBs/1  "Pout"
  Relational/1 -> delta_2/1(In1), RFD/1  "Valid"
  Clk/1 -> Delay3/1
  26_MSBs/1 -> Convert/1
  Convert/1 -> Register/1
  delta_2/1(Out1) -> Delay1/1, Register/2, Register1/2
  Register/1 -> Par_26/1
  Delay2/1 -> Serial2Par/1(Sin)
  Delay3/1 -> delta_1/1(In1)
  6_LSBs/1 -> Register1/1
  Register1/1 -> Address_6/1
  Logical/1 -> Valid/1
  Delay1/1 -> Logical/1
  nRST/1 -> Logical/2, Inverter/1
  Inverter/1 -> Logical1/2, Counter/1
  Logical1/1 -> Counter/2

== system Xcvr_SSB_AM_2p5/TX Filters I=8192/Commutator ==
  Yn1 : Inport
  Yn2 : Inport  Port=2
  Constant : xbsIndex_r4/Constant  const=32  gui_display_data_type=Fixed-point  arith_type=Unsigned  n_bits=7  bin_pt=0  preci_type=Single  exp_width=8  frac_width=24  explicit_period=off  period=1  equ=P=C  opselect=C  inp2=PCIN>>17  opr=+  inp1=P  carry=CIN  dbl_ovrd=off  block_type=constant
      settings: block_version=9.2.00
  Constant1 : xbsIndex_r4/Constant  const=64  gui_display_data_type=Fixed-point  arith_type=Unsigned  n_bits=7  bin_pt=0  preci_type=Single  exp_width=8  frac_width=24  explicit_period=off  period=1  equ=P=C  opselect=C  inp2=PCIN>>17  opr=+  inp1=P  carry=CIN  dbl_ovrd=off  block_type=constant
      settings: block_version=9.2.00
  Convert : xbsIndex_r4/Convert  gui_display_data_type=Fixed-point  arith_type="Signed  (2's comp)"  n_bits=14  bin_pt=13  float_type=Single  exp_bits=8  fraction_bits=24  quantization="Round  (unbiased: +/- Inf)"  overflow=Saturate  en=off  latency=0  dbl_ovrd=off  pipeline=off  block_type=convert
      settings: block_version=12.2
  Convert1 : xbsIndex_r4/Convert  gui_display_data_type=Fixed-point  arith_type="Signed  (2's comp)"  n_bits=14  bin_pt=13  float_type=Single  exp_bits=8  fraction_bits=24  quantization="Round  (unbiased: +/- Inf)"  overflow=Saturate  en=off  latency=0  dbl_ovrd=off  pipeline=off  block_type=convert
      settings: block_version=12.2
  Counter : xbsIndex_r4/Counter  cnt_type=Free Running  cnt_to=Inf  operation=Up  start_count=0  cnt_by_val=1  arith_type=Unsigned  n_bits=7  bin_pt=0  load_pin=off  rst=off  en=off  explicit_period=on  period=1/Fs  dbl_ovrd=off  use_behavioral_HDL=off  implementation=Fabric  use_rpm=off  block_type=counter
      settings: block_version=9.2.00
  Counter1 : xbsIndex_r4/Counter  cnt_type=Free Running  cnt_to=Inf  operation=Up  start_count=0  cnt_by_val=1  arith_type=Unsigned  n_bits=1  bin_pt=0  load_pin=off  rst=off  en=off  explicit_period=on  period=64/Fs  dbl_ovrd=off  use_behavioral_HDL=off  implementation=Fabric  use_rpm=off  block_type=counter
      settings: block_version=9.2.00
  Down Sample{1..4} (4 alike) : xbsIndex_r4/Down Sample  sample_ratio=128  sample_phase="Last Value of Frame  (most efficient)"  en=off  latency=1  dbl_ovrd=off  block_type=dsamp
      settings: block_version=9.2.00
  Mux : xbsIndex_r4/Mux  inputs=2  en=off  latency=1  precision=Full  arith_type=Unsigned  n_bits=16  bin_pt=14  quantization=Truncate  overflow=Wrap  dbl_ovrd=off  block_type=mux
      settings: block_version=9.2.00
  Mux1 : xbsIndex_r4/Mux  inputs=2  en=off  latency=1  precision=Full  arith_type=Unsigned  n_bits=16  bin_pt=14  quantization=Truncate  overflow=Wrap  dbl_ovrd=off  block_type=mux
      settings: block_version=9.2.00
  Register{,1..3} (4 alike) : xbsIndex_r4/Register  init=0  rst=off  en=on  dbl_ovrd=off  block_type=register
      settings: block_version=9.2.00
  Reinterpret : xbsIndex_r4/Reinterpret  force_arith_type=on  arith_type="Signed  (2's comp)"  force_bin_pt=on  bin_pt=15  block_type=reinterpret
      settings: infoedit="Changes signal type without altering the binary representation.   You can changed the signal between signed and unsigned, and relocate the binary point.<P><P>Hardware notes: In hardware this block costs nothing.<P><P>Example:  Suppose the input is 6 bits wide, signed, with 2 fractional bits, and the output is forced to unsigned with 0 fractional bits.  Then an input of -2.0 (1110.00 in binary 2's complement) becomes an output of 56 (111000 in binary)."  block_version=9.2.00
  Reinterpret1 : xbsIndex_r4/Reinterpret  force_arith_type=on  arith_type="Signed  (2's comp)"  force_bin_pt=on  bin_pt=15  block_type=reinterpret
      settings: infoedit="Changes signal type without altering the binary representation.   You can changed the signal between signed and unsigned, and relocate the binary point.<P><P>Hardware notes: In hardware this block costs nothing.<P><P>Example:  Suppose the input is 6 bits wide, signed, with 2 fractional bits, and the output is forced to unsigned with 0 fractional bits.  Then an input of -2.0 (1110.00 in binary 2's complement) becomes an output of 56 (111000 in binary)."  block_version=9.2.00
  Relational : xbsIndex_r4/Relational  mode=a=b  en=off  latency=1  dbl_ovrd=off  block_type=relational
      settings: block_version=9.2.00
  Relational1 : xbsIndex_r4/Relational  mode=a=b  en=off  latency=1  dbl_ovrd=off  block_type=relational
      settings: block_version=9.2.00
  Shift : xbsIndex_r4/Shift  shift_dir=Left  shift_bits=1  en=off  latency=0  precision=Full  arith_type="Signed  (2's comp)"  n_bits=16  bin_pt=14  quantization=Truncate  overflow=Wrap  dbl_ovrd=off  block_type=shift
      settings: block_version=12.2
  Shift1 : xbsIndex_r4/Shift  shift_dir=Left  shift_bits=1  en=off  latency=0  precision=Full  arith_type="Signed  (2's comp)"  n_bits=16  bin_pt=14  quantization=Truncate  overflow=Wrap  dbl_ovrd=off  block_type=shift
      settings: block_version=12.2
  Real : Outport
  Imag : Outport  Port=2
  wires:
  Yn2/1 -> Register2/1, Register3/1
  Yn1/1 -> Register1/1, Register/1
  Counter/1 -> Relational/1, Relational1/1
  Relational/1 -> Register/2, Register2/2
  Constant/1 -> Relational/2
  Register/1 -> Down Sample2/1
  Constant1/1 -> Relational1/2
  Relational1/1 -> Register1/2, Register3/2
  Register1/1 -> Down Sample1/1
  Register2/1 -> Down Sample3/1
  Down Sample2/1 -> Mux/2
  Down Sample3/1 -> Mux/3
  Counter1/1 -> Mux/1, Mux1/1
  Register3/1 -> Down Sample4/1
  Down Sample4/1 -> Mux1/3
  Mux/1 -> Reinterpret/1
  Down Sample1/1 -> Mux1/2
  Mux1/1 -> Reinterpret1/1
  Reinterpret/1 -> Shift/1
  Reinterpret1/1 -> Shift1/1
  Shift/1 -> Convert/1
  Convert/1 -> Real/1
  Shift1/1 -> Convert1/1
  Convert1/1 -> Imag/1
